simulink model "verify_Inverter_mdl"  (R2016b)
settings: Solver=ode45  StartTime=0.0  StopTime=15  MaxStep=1  RelTol=1e-3  EnableMultiTasking=on
libraries: carnot x1, simulink x1
settings Model: Creator=drhf  LastModifiedBy=drhf
settings DataIOCC: SaveFormat=Array  SignalLoggingSaveFormat=ModelDataLogs
settings OptimizationCC: ExpressionDepthLimit=2147483647  LifeSpan=inf
settings DebuggingCC: UnderspecifiedInitializationDetection=Classic  MergeDetectMultiDrivingBlocksExec=none  SolverPrmCheckMsg=warning  FcnCallInpInsideContextMsg=warning  StateNameClashWarn=warning  SFUnexpectedBacktrackingDiag=warning  SFNoUnconditionalDefaultTransitionDiag=warning  SFExecutionAtInitializationDiag=none
settings HardwareCC: ProdBitPerPointer=32  ProdBitPerSizeT=32  ProdBitPerPtrDiffT=32  ProdLargestAtomicFloat=None  ProdIntDivRoundTo=Undefined  ProdEndianess=Unspecified  ProdWordSize=32  ProdHWDeviceType=32-bit Generic
settings ModelReferenceCC: PropagateSignalLabelsOutOfModel=off
settings GRTTargetCC: TargetLangStandard=C89/C90 (ANSI)  GeneratePreprocessorConditionals=Disable all  CombineOutputUpdateFcns=off  GRTInterface=on
settings ConfigComp: CovMetricSettings=dw  CovHtmlReporting=on  CovSaveCumulativeToWorkspaceVar=on  CovSaveSingleToWorkspaceVar=on  CovExternalEMLEnable=off

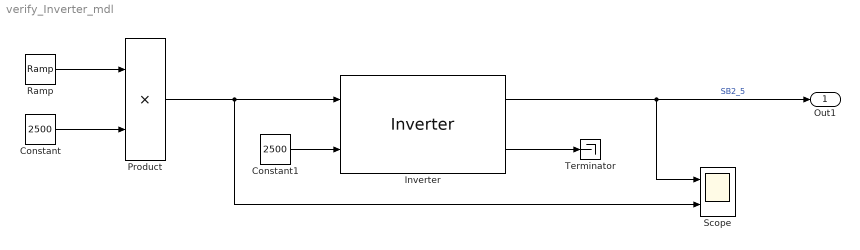
== system verify_Inverter_mdl ==
  Constant : Constant  Value=2500
  Constant1 : Constant  Value=2500
  Inverter : carnot/Source/Electric_Generator/Inverter  P0=5000  ol=1.2  power_steps=[0 0.05 0.1 0.2 0.3 0.5 1 1.2 1.21]  eta_steps=[0 0.924 0.958 0.974 0.979 0.981 0.98 0.95 0.95]  standby=1
  Product : Product
  Ramp : simulink/Sources/Ramp  slope=0.1  start=0  X0=0
  Scope : Scope  NumInputPorts=2
  Terminator : Terminator
  Out1 : Outport
  wires:
  Constant/1 -> Product/2
  Product/1 -> Inverter/1, Scope/2
  Constant1/1 -> Inverter/2
  Inverter/2 -> Terminator/1
  Inverter/1 -> Scope/1, Out1/1  "SB2_5"
  Ramp/1 -> Product/1
